simulink model "control_action_throttle"  (R2023b)
settings: Solver=FixedStepDiscrete  StartTime=0.0  StopTime=9  FixedStep=1e-3  RelTol=1e-3
undefined symbols (not defined in the file or in its folder): MyEnum
libraries: simulink x2
settings Model: Creator=Beshary  LastModifiedBy=Beshary
settings DataIOCC: ExternalInput=[t, Thtottle_Position_Senor_1,Thtottle_Position_Senor_2,Thtottle_Position_Setpoint]  LoadExternalInput=on  SaveFormat=Array

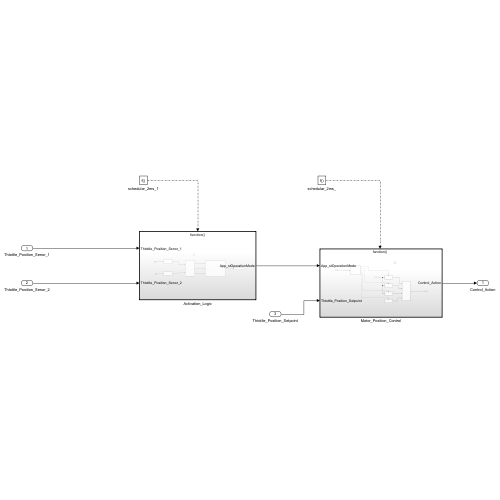
[thumbnail: Simulink's stored preview of the top-level diagram]
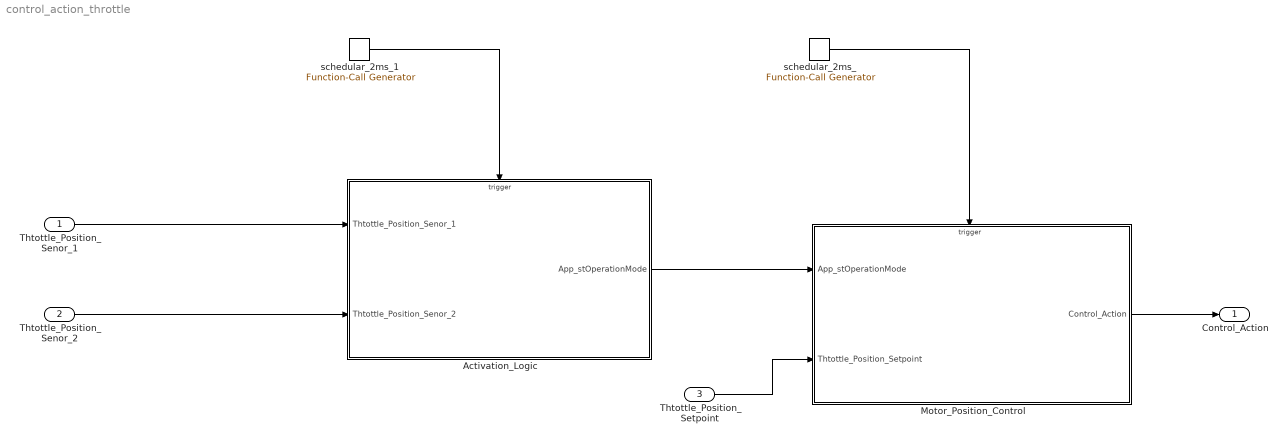
== system control_action_throttle ==
  Thtottle_Position_Senor_1 : Inport
  Thtottle_Position_Senor_2 : Inport  Port=2
  Thtottle_Position_Setpoint : Inport  Port=3
  Activation_Logic : Subsystem
  Motor_Position_Control : Subsystem
  schedular_2ms_ : simulink/Ports & Subsystems/Function-Call Generator  sample_time=2  numberOfIterations=1  DisallowWideOutput=off
  schedular_2ms_1 : simulink/Ports & Subsystems/Function-Call Generator  sample_time=2  numberOfIterations=1  DisallowWideOutput=off
  Control_Action : Outport
  wires:
  Thtottle_Position_Senor_1/1 -> Activation_Logic/1(Thtottle_Position_Senor_1)
  Activation_Logic/1(App_stOperationMode) -> Motor_Position_Control/1(App_stOperationMode)
  schedular_2ms_1/1 -> Activation_Logic/Trigger
  Motor_Position_Control/1(Control_Action) -> Control_Action/1
  Thtottle_Position_Senor_2/1 -> Activation_Logic/2(Thtottle_Position_Senor_2)
  Thtottle_Position_Setpoint/1 -> Motor_Position_Control/2(Thtottle_Position_Setpoint)
  schedular_2ms_/1 -> Motor_Position_Control/Trigger

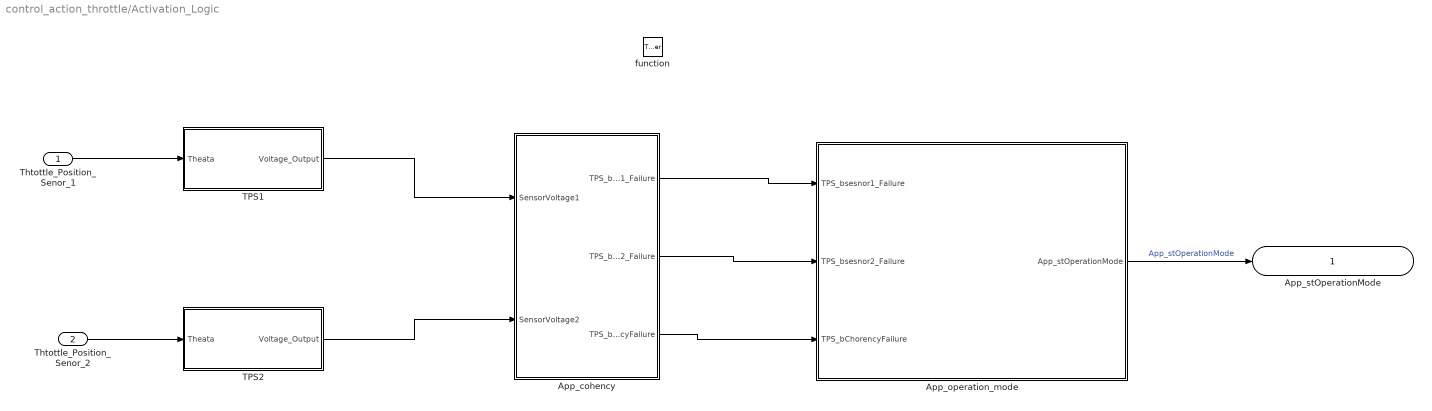
== system control_action_throttle/Activation_Logic ==
  Thtottle_Position_Senor_1 : Inport
  Thtottle_Position_Senor_2 : Inport  Port=2
  function : TriggerPort  TriggerType=function-call  VariantControl=(inherit)
  App_cohency : Subsystem
  App_operation_mode : Subsystem
  TPS1 : Subsystem
  TPS2 : Subsystem
  App_stOperationMode : Outport
  wires:
  App_operation_mode/1(App_stOperationMode) -> App_stOperationMode/1  "App_stOperationMode"
  TPS1/1(Voltage_Output) -> App_cohency/1(SensorVoltage1)
  TPS2/1(Voltage_Output) -> App_cohency/2(SensorVoltage2)
  Thtottle_Position_Senor_1/1 -> TPS1/1(Theata)
  App_cohency/3(TPS_bChorencyFailure) -> App_operation_mode/3(TPS_bChorencyFailure)
  App_cohency/2(TPS_bsesnor2_Failure) -> App_operation_mode/2(TPS_bsesnor2_Failure)
  App_cohency/1(TPS_bsesnor1_Failure) -> App_operation_mode/1(TPS_bsesnor1_Failure)
  Thtottle_Position_Senor_2/1 -> TPS2/1(Theata)

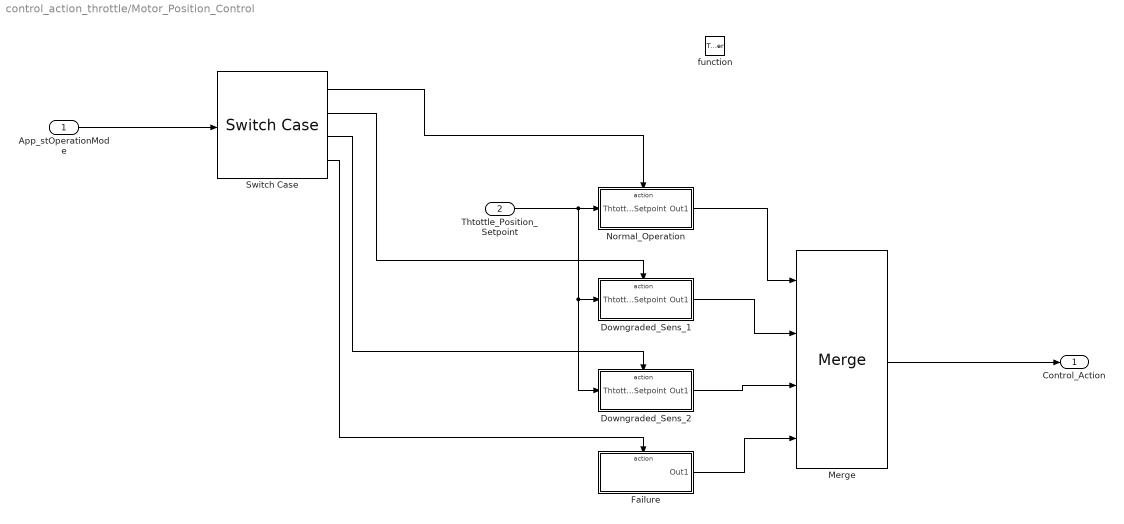
== system control_action_throttle/Motor_Position_Control ==
  App_stOperationMode : Inport
  Thtottle_Position_Setpoint : Inport  Port=2
  function : TriggerPort  TriggerType=function-call  VariantControl=(inherit)
  Downgraded_Sens_1 : Subsystem  TreatAsAtomicUnit=on
  Downgraded_Sens_2 : Subsystem  TreatAsAtomicUnit=on
  Failure : Subsystem  TreatAsAtomicUnit=on
  Merge : Merge  Inputs=4
  Normal_Operation : Subsystem  TreatAsAtomicUnit=on
  Switch Case : SwitchCase  CaseConditions={MyEnum.Normal,MyEnum.DowngradedS1,MyEnum.DowngradedS2,MyEnum.Failure}  ShowDefaultCase=off
  Control_Action : Outport
  wires:
  App_stOperationMode/1 -> Switch Case/1
  Switch Case/1 -> Normal_Operation/Action
  Normal_Operation/1(Out1) -> Merge/1
  Downgraded_Sens_1/1(Out1) -> Merge/2
  Downgraded_Sens_2/1(Out1) -> Merge/3
  Failure/1(Out1) -> Merge/4
  Thtottle_Position_Setpoint/1 -> Downgraded_Sens_2/1(Thtottle_Position_Setpoint), Downgraded_Sens_1/1(Thtottle_Position_Setpoint), Normal_Operation/1(Thtottle_Position_Setpoint)
  Switch Case/2 -> Downgraded_Sens_1/Action
  Switch Case/3 -> Downgraded_Sens_2/Action
  Switch Case/4 -> Failure/Action
  Merge/1 -> Control_Action/1

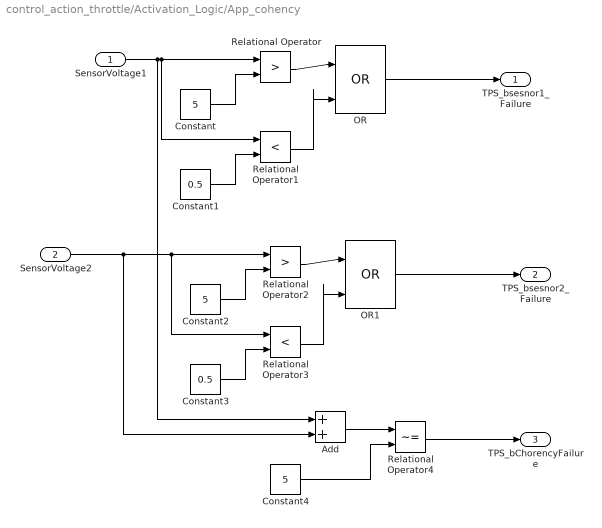
== system control_action_throttle/Activation_Logic/App_cohency ==
  SensorVoltage1 : Inport
  SensorVoltage2 : Inport  Port=2
  Add : Sum
  Constant : Constant  Value=5
  Constant1 : Constant  Value=0.5
  Constant2 : Constant  Value=5
  Constant3 : Constant  Value=0.5
  Constant4 : Constant  Value=5
  OR : Logic  Operator=OR  IconShape=distinctive  AllPortsSameDT=off  OutDataTypeStr=boolean
  OR1 : Logic  Operator=OR  IconShape=distinctive  AllPortsSameDT=off  OutDataTypeStr=boolean
  Relational Operator : RelationalOperator  Operator=>  OutDataTypeStr=boolean  RndMeth=Simplest  InputSameDT=off
  Relational Operator1 : RelationalOperator  Operator=<  OutDataTypeStr=boolean  RndMeth=Simplest  InputSameDT=off
  Relational Operator2 : RelationalOperator  Operator=>  OutDataTypeStr=boolean  RndMeth=Simplest  InputSameDT=off
  Relational Operator3 : RelationalOperator  Operator=<  OutDataTypeStr=boolean  RndMeth=Simplest  InputSameDT=off
  Relational Operator4 : RelationalOperator  Operator=~=  OutDataTypeStr=boolean  RndMeth=Simplest  InputSameDT=off
  TPS_bsesnor1_Failure : Outport
  TPS_bsesnor2_Failure : Outport  Port=2
  TPS_bChorencyFailure : Outport  Port=3
  wires:
  Constant/1 -> Relational Operator/2
  Relational Operator/1 -> OR/1
  Constant1/1 -> Relational Operator1/2
  SensorVoltage1/1 -> Add/1, Relational Operator1/1, Relational Operator/1
  Relational Operator1/1 -> OR/2
  OR/1 -> TPS_bsesnor1_Failure/1
  Relational Operator3/1 -> OR1/2
  SensorVoltage2/1 -> Add/2, Relational Operator2/1, Relational Operator3/1
  Constant3/1 -> Relational Operator3/2
  Relational Operator2/1 -> OR1/1
  Constant2/1 -> Relational Operator2/2
  OR1/1 -> TPS_bsesnor2_Failure/1
  Add/1 -> Relational Operator4/1
  Constant4/1 -> Relational Operator4/2
  Relational Operator4/1 -> TPS_bChorencyFailure/1

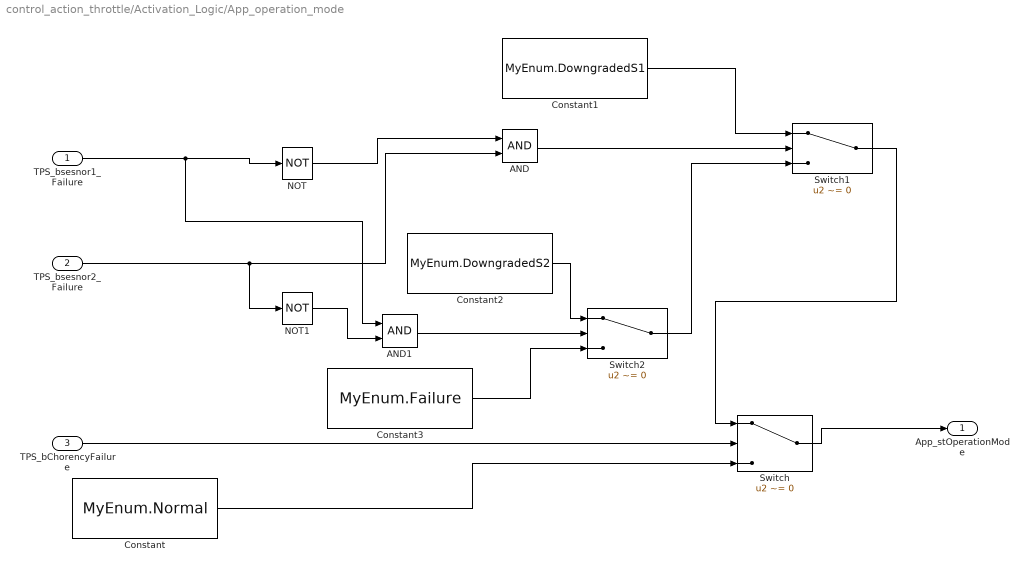
== system control_action_throttle/Activation_Logic/App_operation_mode ==
  TPS_bsesnor1_Failure : Inport
  TPS_bsesnor2_Failure : Inport  Port=2
  TPS_bChorencyFailure : Inport  Port=3
  AND : Logic  AllPortsSameDT=off  OutDataTypeStr=boolean
  AND1 : Logic  AllPortsSameDT=off  OutDataTypeStr=boolean
  Constant : Constant  Value=MyEnum.Normal
  Constant1 : Constant  Value=MyEnum.DowngradedS1
  Constant2 : Constant  Value=MyEnum.DowngradedS2
  Constant3 : Constant  Value=MyEnum.Failure
  NOT : Logic  Operator=NOT  IconShape=distinctive  AllPortsSameDT=off  OutDataTypeStr=boolean
  NOT1 : Logic  Operator=NOT  IconShape=distinctive  AllPortsSameDT=off  OutDataTypeStr=boolean
  Switch : Switch  Criteria=u2 ~= 0  SaturateOnIntegerOverflow=off  InputSameDT=off
  Switch1 : Switch  Criteria=u2 ~= 0  SaturateOnIntegerOverflow=off  InputSameDT=off
  Switch2 : Switch  Criteria=u2 ~= 0  SaturateOnIntegerOverflow=off  InputSameDT=off
  App_stOperationMode : Outport  OutDataTypeStr=Enum: MyEnum
  wires:
  TPS_bChorencyFailure/1 -> Switch/2
  Constant/1 -> Switch/3
  Switch/1 -> App_stOperationMode/1
  TPS_bsesnor1_Failure/1 -> AND1/1, NOT/1
  NOT/1 -> AND/1
  TPS_bsesnor2_Failure/1 -> NOT1/1, AND/2
  AND/1 -> Switch1/2
  Switch1/1 -> Switch/1
  Constant1/1 -> Switch1/1
  NOT1/1 -> AND1/2
  AND1/1 -> Switch2/2
  Constant2/1 -> Switch2/1
  Constant3/1 -> Switch2/3
  Switch2/1 -> Switch1/3

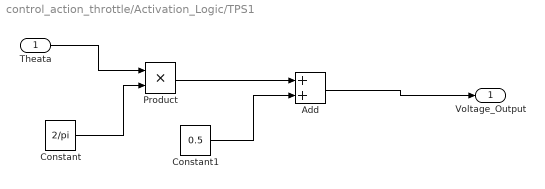
== system control_action_throttle/Activation_Logic/TPS1 ==
  Theata : Inport
  Add : Sum
  Constant : Constant  Value=2/pi
  Constant1 : Constant  Value=0.5
  Product : Product
  Voltage_Output : Outport
  wires:
  Constant/1 -> Product/2
  Product/1 -> Add/1
  Theata/1 -> Product/1
  Constant1/1 -> Add/2
  Add/1 -> Voltage_Output/1

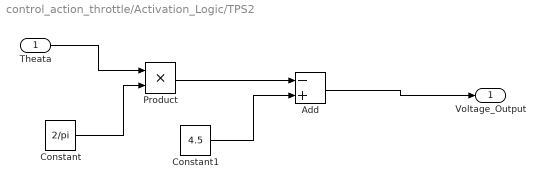
== system control_action_throttle/Activation_Logic/TPS2 ==
  Theata : Inport
  Add : Sum  Inputs=-+
  Constant : Constant  Value=2/pi
  Constant1 : Constant  Value=4.5
  Product : Product
  Voltage_Output : Outport
  wires:
  Add/1 -> Voltage_Output/1
  Constant1/1 -> Add/2
  Theata/1 -> Product/1
  Product/1 -> Add/1
  Constant/1 -> Product/2

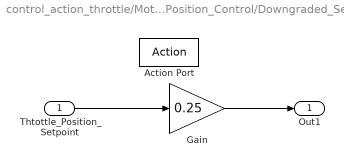
== system control_action_throttle/Motor_Position_Control/Downgraded_Sens_1 ==
  Thtottle_Position_Setpoint : Inport
  Action Port : ActionPort  ActionPortLabel=case [ DowngradedS1 ]:
  Gain : Gain  Gain=0.25
  Out1 : Outport
  wires:
  Thtottle_Position_Setpoint/1 -> Gain/1
  Gain/1 -> Out1/1

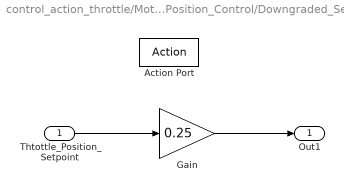
== system control_action_throttle/Motor_Position_Control/Downgraded_Sens_2 ==
  Thtottle_Position_Setpoint : Inport
  Action Port : ActionPort  ActionPortLabel=case [ DowngradedS2 ]:
  Gain : Gain  Gain=0.25
  Out1 : Outport
  wires:
  Thtottle_Position_Setpoint/1 -> Gain/1
  Gain/1 -> Out1/1

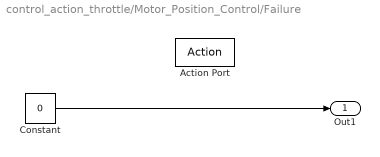
== system control_action_throttle/Motor_Position_Control/Failure ==
  Action Port : ActionPort  ActionPortLabel=case [ Failure ]:
  Constant : Constant  Value=0
  Out1 : Outport
  wires:
  Constant/1 -> Out1/1

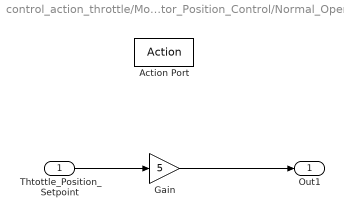
== system control_action_throttle/Motor_Position_Control/Normal_Operation ==
  Thtottle_Position_Setpoint : Inport
  Action Port : ActionPort  ActionPortLabel=case [ Normal ]:
  Gain : Gain  Gain=5
  Out1 : Outport
  wires:
  Thtottle_Position_Setpoint/1 -> Gain/1
  Gain/1 -> Out1/1
